simulink model "Problem_2"  (R2020a)
settings: Solver=VariableStepAuto  StartTime=0.0  StopTime=10.0  RelTol=1e-3
settings Model: Creator=user  LastModifiedBy=user

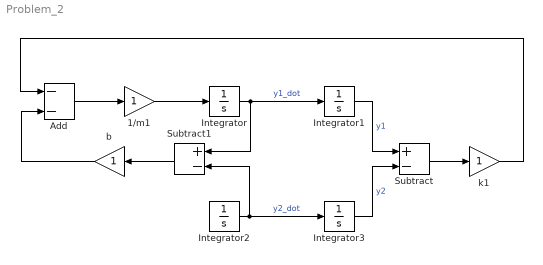
== system Problem_2 ==
  1/m1 : Gain
  Add : Sum  Inputs=--
  Integrator{,1..3} (4 alike) : Integrator
  Subtract : Sum  Inputs=+-
  Subtract1 : Sum  Inputs=+-
  b : Gain
  k1 : Gain
  wires:
  Integrator/1 -> Subtract1/1, Integrator1/1  "y1_dot"
  Integrator2/1 -> Integrator3/1, Subtract1/2  "y2_dot"
  Integrator1/1 -> Subtract/1  "y1"
  Integrator3/1 -> Subtract/2  "y2"
  Subtract/1 -> k1/1
  1/m1/1 -> Integrator/1
  Add/1 -> 1/m1/1
  k1/1 -> Add/1
  Subtract1/1 -> b/1
  b/1 -> Add/2
